simulink model "AGTF30SysDyn_PExPIn"  (R2023b)
settings: Solver=ode4  StartTime=0.0  StopTime=MWS.In.tend  FixedStep=MWS.In.Ts  RelTol=1e-3  EnableMultiTasking=on
model workspace: external: MAT-File (data not in the file)
values from neighbouring files (symbols this model uses):
  MWS = setup_initialize(MWS,startPt,SSsolverSP)    [Setup_Simulation.m]    (also in run_AGTF30e_script.m = Setup_Simulation(inputMethod,MWS.In,filename,Mdl,SSsolverSP))
undefined symbols (not defined in the file or in its folder): DiscIntNeverNeededParam
libraries: simulink x32, Lib_Solve_ModelSource_TMATS x28, Lib_EMTAT x27, Lib_Cntrl_FirstOrderSensor_TMATS x19, Lib_Cntrl_FirstOrderActuator_TMATS x2, Lib_Cntrl_LimitSelect_TMATS x2, Lib_Solve_OuterLoopIntegrator_TMATS x2, Lib_Cntrl_CorrectedSpeed_TMATS x1, Lib_Solve_IterNRSolverJC_TMATS x1, slpidlib x1
(part 4 of 8)

== system AGTF30SysDyn_PExPIn/Control System/Wf Controller/Controller/Set-Points ==
  Nominal SP : Inport
  N1cSP Limit SPs : Inport  Port=2
  Wf Limit SPs : Inport  Port=3
  Bus Creator : BusCreator  Inputs=3
  Bus Creator1 : BusCreator  Inputs=7
  Bus Creator2 : BusCreator  Inputs=3
  Demux : Demux  Outputs=7
  Demux1 : Demux  Outputs=3
  SPs : Outport  VectorParamsAs1DForOutWhenUnconnected=off
  wires:
  Nominal SP/1 -> Bus Creator/1  "N1c"
  N1cSP Limit SPs/1 -> Demux/1
  Bus Creator/1 -> SPs/1
  Demux/1 -> Bus Creator1/1  "T3Max"
  Demux/2 -> Bus Creator1/2  "T4Max"
  Demux/3 -> Bus Creator1/3  "T45Max"
  Demux/4 -> Bus Creator1/4  "N1Max"
  Demux/5 -> Bus Creator1/5  "N3Max"
  Demux/6 -> Bus Creator1/6  "Ps3Max"
  Demux/7 -> Bus Creator1/7  "Ps3Min"
  Bus Creator1/1 -> Bus Creator/2  "N1cSPLims"
  Bus Creator2/1 -> Bus Creator/3  "WfLims"
  Demux1/1 -> Bus Creator2/1  "Accel"
  Demux1/2 -> Bus Creator2/2  "Decel"
  Demux1/3 -> Bus Creator2/3  "WfMin"
  Wf Limit SPs/1 -> Demux1/1

== system AGTF30SysDyn_PExPIn/Control System/Wf Controller/Controller/Wf Limit Controllers ==
  note: ENABLE MIN FUEL FLOW LIMIT WHEN DECEL LIMIT IS NOT IN USE
  Alt : Inport
  MN : Inport  Port=2
  Wfmin : Inport  Port=3
  Wfmax : Inport  Port=4
  Wfcmd : Inport  Port=5
  phiEPT : Inport  Port=6
  phiBoost : Inport  Port=7
  N1cN : Inport  Port=8
  ps3 : Inport  Port=9
  RegNum : Inport  Port=10
  Accel Controller : Subsystem
  Compare To Constant : simulink/Logic and Bit Operations/Compare To Constant  relop=~=  const=7  OutDataTypeStr=boolean
  Decel Controller : Subsystem
  Divide : Product  Inputs=**
  Gain : Gain  Gain=0.95
  Memory : Memory
  Mux : Mux  Inputs=3
  Wf Accel : Outport  VectorParamsAs1DForOutWhenUnconnected=off
  Wf Decel : Outport  Port=2  VectorParamsAs1DForOutWhenUnconnected=off
  Wf Min : Outport  Port=3  VectorParamsAs1DForOutWhenUnconnected=off
  SPs : Outport  Port=4  VectorParamsAs1DForOutWhenUnconnected=off
  wires:
  Alt/1 -> Decel Controller/1(Alt), Accel Controller/1(Alt)
  Wfmax/1 -> Accel Controller/6(Wfmax)
  Decel Controller/2(WfminDecel_SP) -> Mux/2  "WfMinDecel"
  Accel Controller/2(WfmaxAccel_SP) -> Mux/1  "WfMaxAccel"
  Wfcmd/1 -> Accel Controller/7(Wfcmd), Decel Controller/7(Wf)
  Wfmin/1 -> Gain/1, Decel Controller/6(Wfmin)
  Decel Controller/1(Wfdmd) -> Wf Decel/1
  Accel Controller/1(Wfdmd) -> Wf Accel/1
  Mux/1 -> SPs/1
  MN/1 -> Decel Controller/2(MN), Accel Controller/2(MN)
  phiEPT/1 -> Decel Controller/4(phiEPT), Accel Controller/4(phiEPT)
  phiBoost/1 -> Decel Controller/5(phiBoost), Accel Controller/5(phiBoost)
  ps3/1 -> Accel Controller/8(ps3), Decel Controller/8(ps3)
  N1cN/1 -> Decel Controller/3(N1cN), Accel Controller/3(N1cN)
  Gain/1 -> Divide/1  "WfMin"
  Compare To Constant/1 -> Divide/2
  Divide/1 -> Mux/3, Wf Min/1
  RegNum/1 -> Memory/1
  Memory/1 -> Compare To Constant/1

== system AGTF30SysDyn_PExPIn/Control System/Wf Controller/Controller/Wf Limit Select ==
  WfReq : Inport
  Limits : Inport  Port=2
  Limit Selection : Lib_Cntrl_LimitSelect_TMATS/Limit Selection  SelectVec_M=MWS.Cntrl.WfCntrl.WfLim.Type  LimitsEn_M=MWS.Cntrl.WfCntrl.WfLim.En
  Wfdmd : Outport  VectorParamsAs1DForOutWhenUnconnected=off
  RegNum : Outport  Port=2  VectorParamsAs1DForOutWhenUnconnected=off
  wires:
  WfReq/1 -> Limit Selection/1
  Limits/1 -> Limit Selection/2
  Limit Selection/1 -> Wfdmd/1
  Limit Selection/2 -> RegNum/1

== system AGTF30SysDyn_PExPIn/EngineSystem/Power System/Electrical Power System/EM Variant Subsystem ==
  Vs [V] : Inport
  NemL [rpm] : Inport  Port=2
  TrqEML [ft-lb] : Inport  Port=3
  NemH [rpm] : Inport  Port=4
  TrqEMH [ft-lb] : Inport  Port=5
  NemS [rpm] : Inport  Port=6
  TrqEMS [ft-lb] : Inport  Port=7
  NemR [rpm] : Inport  Port=8
  TrqEMR [ft-lb] : Inport  Port=9
  NemC [rpm] : Inport  Port=10
  TrqEMC [ft-lb] : Inport  Port=11
  NemP [rpm] : Inport  Port=12
  TrqEMP [ft-lb] : Inport  Port=13
  Scalar DEM Subsystem : Subsystem  VariantControl=MWS.In.Options.EngineEMInt == 1
  Scalar PGB EM Subsystem : Subsystem  VariantControl=MWS.In.Options.EngineEMInt == 2
  Io [A] : Outport
  Out_LPEMbranch : Outport  Port=2
  Out_HPEMbranch : Outport  Port=3
  Out_SEMbranch : Outport  Port=4
  Out_REMbranch : Outport  Port=5
  Out_CEMbranch : Outport  Port=6
  Out_PEMbranch : Outport  Port=7

== system AGTF30SysDyn_PExPIn/EngineSystem/Power System/Electrical Power System/Energy Storage Subsystem ==
  I_2 [A] : Inport
  Load [hp] : Inport  Port=2
  Bus Creator : BusCreator  Inputs=9
  Bus Selector : BusSelector  OutputSignals=P_1; W,P_2; W
  Bus Selector1 : BusSelector  OutputSignals=P_2; W,I; A
  Bus Selector2 : BusSelector  OutputSignals=I; A
  Cable : Lib_EMTAT/Components/Power Flow/Cable  R=MWS.EPS.Cable.R
      settings: AttributesFormatString=Cable  SourceProductName=EMTAT
  Constant1 : Constant  Value=0
  Constant2 : Constant  Value=0
  Current Junction : Lib_EMTAT/Components/Power Flow/Current Junction  Nb=1
      settings: AttributesFormatString=Current Junction  SourceProductName=EMTAT
  Current Junction1 : Lib_EMTAT/Components/Power Flow/Current Junction  Nb=1
      settings: AttributesFormatString=Current Junction  SourceProductName=EMTAT
  DCDC Variant Subsystem : Subsystem  Variant=on
  ESD Variant Subsystem : Subsystem  Variant=on
  Mux : Mux  Inputs=2
  Resistive Load Bank : Lib_EMTAT/Components/Power Flow/Resistive Load Bank
      settings: AttributesFormatString=Resistive Load Bank  SourceProductName=EMTAT
  Sum1 : Sum  Inputs=+|+
  Terminator1 : Terminator
  Terminator2 : Terminator
  Unit Delay : UnitDelay  InitialCondition=MWS.EPS.Cable.Iout_IC  SampleTime=-1  HasFrameUpgradeWarning=on
  hp to W : Gain  Gain=745.7
  V_DC_Out [V] : Outport
  Out_SupplySys : Outport  Port=2
  SoC [%] : Outport  Port=3
  wires:
  Sum1/1 -> [ESD_Pwr]
  Bus Selector1/1 -> [SuppCable_Pwr], Sum1/1  "<P_2; W>"
  Unit Delay/1 -> Cable/4
  Bus Selector/2 -> [DCDC_Pwr]  "<P_2; W>"
  Cable/1 -> DCDC Variant Subsystem/1(V_ESD [V])
  ESD Variant Subsystem/2(SoC [%]) -> SoC [%]/1
  Load [hp]/1 -> hp to W/1
  DCDC Variant Subsystem/3(Outputs) -> Bus Selector/1
  I_2 [A]/1 -> Current Junction1/1, Mux/1
  Bus Selector/1 -> [Bus_Pwr]  "<P_1; W>"
  Cable/3 -> Terminator1/1
  Cable/5 -> Unit Delay/1
  Constant1/1 -> Cable/3
  DCDC Variant Subsystem/2(Vo [V]) -> [V_Bus], V_DC_Out [V]/1, Resistive Load Bank/1
  Cable/2 -> Bus Selector1/1
  Bus Creator/1 -> Out_SupplySys/1
  [DCDC_Pwr] -> Bus Creator/2  "DCDC_Pwr"
  [Bus_Pwr] -> Bus Creator/1  "Bus_Pwr"
  [ESD_Pwr] -> Bus Creator/4  "ESD_Pwr"
  [SuppCable_Pwr] -> Bus Creator/3  "SuppCable_Pwr"
  DCDC Variant Subsystem/1(Io [A]) -> Cable/2
  Cable/4 -> ESD Variant Subsystem/1(I [A])
  ESD Variant Subsystem/1(Vo [V]) -> [V_ESD], Cable/1
  Resistive Load Bank/3 -> Mux/2
  Resistive Load Bank/1 -> Bus Selector2/1
  Resistive Load Bank/2 -> Terminator2/1
  Constant2/1 -> Resistive Load Bank/3
  Mux/1 -> Current Junction/1
  Current Junction/1 -> DCDC Variant Subsystem/2(I_Bus [A])
  hp to W/1 -> Sum1/2, Resistive Load Bank/2
  Bus Selector1/2 -> [I_ESD]  "<I; A>"
  Bus Selector2/1 -> [I_Load]  "<I; A>"
  [V_Bus] -> Bus Creator/5  "V_Bus"
  [V_ESD] -> Bus Creator/6  "V_ESD"
  [I_Bus] -> Bus Creator/7  "I_Bus"
  [I_Load] -> Bus Creator/8  "I_Load"
  [I_ESD] -> Bus Creator/9  "I_ESD"
  Current Junction1/1 -> [I_Bus]

== system AGTF30SysDyn_PExPIn/Control System/Electric Machine Controllers/EM Controllers/DEM Control/DEM EM Controllers ==
  note: The load is the electrical power demand from the bus needed for sustaining engine and aircraft subsystems (PExAC) and extraneous propulsive loads (in the case of PEx mode). In the case of PEx mode, the electrical load is modified to essentially match the power extraction commanded for the electric machines. "Essentially" is used because it won't match actually given cable losses. So the SOC controller will need to make up a slight difference.
  PwrInLPEMNomMan : Inport
  PwrInLPEMNomManEn : Inport  Port=2
  PwrInLPEMOffNomMan : Inport  Port=3
  PwrInLPEMOffNomManEn : Inport  Port=4
  PwrInHPEMNomMan : Inport  Port=5
  PwrInHPEMNomManEn : Inport  Port=6
  PwrInHPEMOffNomMan : Inport  Port=7
  PwrInHPEMOffNomManEn : Inport  Port=8
  PwrInLP_Base : Inport  Port=9
  PwrInHP_Base : Inport  Port=10
  NemL : Inport  Port=11
  NemH : Inport  Port=12
  PwrEPT : Inport  Port=13
  PwrInAccel_TEEM : Inport  Port=14
  PwrExAccel_TEEM : Inport  Port=15
  PwrXDecel_TEEM : Inport  Port=16
  PwrCharge : Inport  Port=17
  PExAC : Inport  Port=18
  PwrSys : Inport  Port=19
  EMH Controller : Subsystem
  EML Controller : Subsystem
  EPT Pwr Calc : Subsystem
  Sum : Sum  Inputs=+|+
  PwrEML : Outport
  PwrEMH : Outport  Port=2
  TrqEML : Outport  Port=3
  TrqEMH : Outport  Port=4
  PwrLoad : Outport  Port=5
  wires:
  NemH/1 -> EMH Controller/6(NemH)
  PwrInAccel_TEEM/1 -> EMH Controller/8(PwrInAccel_TEEM)
  EML Controller/2(TrqEML) -> TrqEML/1
  EMH Controller/2(TrqEMH) -> TrqEMH/1
  PwrInLP_Base/1 -> EML Controller/5(PwrInLP_Base)
  PwrInHP_Base/1 -> EMH Controller/5(PwrInHP_Base)
  PwrInLPEMOffNomManEn/1 -> EML Controller/4(PwrInLPEMOffNomManEn)
  NemL/1 -> EML Controller/6(NemL)
  PwrInLPEMNomMan/1 -> EML Controller/1(PwrInLPEMNomMan)
  PwrInHPEMOffNomMan/1 -> EMH Controller/3(PwrInHPEMOffNomMan)
  PwrInHPEMNomManEn/1 -> EMH Controller/2(PwrInHPEMNomManEn)
  EML Controller/1(PwrEML) -> PwrEML/1
  PwrInLPEMNomManEn/1 -> EML Controller/2(PwrInLPEMNomManEn)
  PwrInHPEMOffNomManEn/1 -> EMH Controller/4(PwrInHPEMOffNomManEn)
  PwrInLPEMOffNomMan/1 -> EML Controller/3(PwrInLPEMOffNomMan)
  PwrInHPEMNomMan/1 -> EMH Controller/1(PwrInHPEMNomMan)
  EMH Controller/1(PwrEMH) -> PwrEMH/1
  PwrXDecel_TEEM/1 -> EMH Controller/9(PwrXDecel_TEEM), EML Controller/9(PwrXDecel_TEEM)
  PwrEPT/1 -> EPT Pwr Calc/1(PwrEPT)
  EPT Pwr Calc/1(PwrEML_EPT) -> EML Controller/7(PwrInLPEPT)
  EPT Pwr Calc/2(PwrEMH_EPT) -> EMH Controller/7(PwrInHPEPT)
  Sum/1 -> PwrLoad/1
  PwrCharge/1 -> EMH Controller/10(PwrCharge)
  PwrExAccel_TEEM/1 -> EML Controller/8(PwrExAccel_TEEM)
  PwrSys/1 -> EMH Controller/11(PwrSys), EML Controller/10(PwrSys)
  PExAC/1 -> EMH Controller/12(PExAC)
  EML Controller/3(PwrLoadL) -> [PwrLoadL]
  EMH Controller/3(PwrLoadEMH) -> [PwrLoadH]
  [PwrLoadL] -> Sum/1
  [PwrLoadH] -> Sum/2

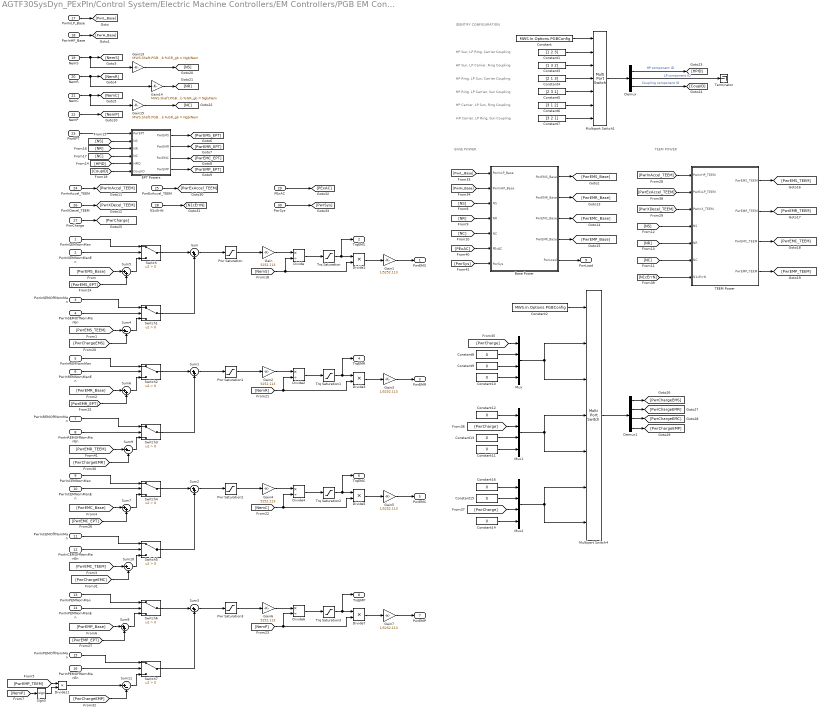
== system AGTF30SysDyn_PExPIn/Control System/Electric Machine Controllers/EM Controllers/PGB EM Control/VEATE EM Controllers ==
  note: HP Sun, LP RIng, Carrier Coupling
  note: HP Sun, LP Carrier, Ring Coupling
  note: IDENTIFY CONFIGURATION
  note: HP Ring, LP Sun, Carrier Coupling
  note: HP Carrier, LP Sun, Ring Coupling
  note: HP Ring, LP Carrier, Sun Coupling
  note: HP Carrier, LP Ring, Sun Coupling
  note: TEEM POWER
  note: BASE POWER
  PwrInSEMNomMan : Inport
  PwrInSEMNomManEn : Inport  Port=2
  PwrInSEMOffNomMan : Inport  Port=3
  PwrInSEMOffNomManEn : Inport  Port=4
  PwrInREMNomMan : Inport  Port=5
  PwrInREMNomManEn : Inport  Port=6
  PwrInREMOffNomMan : Inport  Port=7
  PwrInREMOffNomManEn : Inport  Port=8
  PwrInCEMNomMan : Inport  Port=9
  PwrInCEMNomManEn : Inport  Port=10
  PwrInCEMOffNomMan : Inport  Port=11
  PwrInCEMOffNomManEn : Inport  Port=12
  PwrInPEMNomMan : Inport  Port=13
  PwrInPEMNomManEn : Inport  Port=14
  PwrInPEMOffNomMan : Inport  Port=15
  PwrInPEMOffNomManEn : Inport  Port=16
  PwrInLP_Base : Inport  Port=17
  PwrInHP_Base : Inport  Port=18
  NemS : Inport  Port=19
  NemR : Inport  Port=20
  NemC : Inport  Port=21
  NemP : Inport  Port=22
  PwrEPT : Inport  Port=23
  PwrInAccel_TEEM : Inport  Port=24
  PwrExAccel_TEEM : Inport  Port=25
  PwrXDecel_TEEM : Inport  Port=26
  PwrCharge : Inport  Port=27
  N1cErrN : Inport  Port=28
  PExAC : Inport  Port=29
  PwrSys : Inport  Port=30
  Base Power : Subsystem
  Constant : Constant  Value=MWS.In.Options.PGBConfig
  Constant1 : Constant  Value=[1 2 3]
  Constant{8..16} (9 alike) : Constant  Value=0
  Constant2 : Constant  Value=MWS.In.Options.PGBConfig
  Constant3 : Constant  Value=[1 3 2]
  Constant4 : Constant  Value=[2 1 3]
  Constant5 : Constant  Value=[2 3 1]
  Constant6 : Constant  Value=[3 1 2]
  Constant7 : Constant  Value=[3 2 1]
  Demux : Demux  Outputs=3
  Demux1 : Demux
  Divide{,2,4,6} (4 alike) : Product  Inputs=*/
  Divide{1,3,5,7,11} (5 alike) : Product  Inputs=**
  EPT Powers : Subsystem
  Gain{,2,4,6} (4 alike) : Gain  Gain=5252.113
  Gain{1,3,5,7} (4 alike) : Gain  Gain=1/5252.113
  Gain13 : Gain  Gain=MWS.Shaft.PGB.Sun.GR_gb %GR_gb = Ngb/Nem
  Gain14 : Gain  Gain=MWS.Shaft.PGB.Ring.GR_gb %GR_gb = Ngb/Nem
  Gain15 : Gain  Gain=MWS.Shaft.PGB.Carrier.GR_gb %GR_gb = Ngb/Nem
  Multiport Switch1 : MultiPortSwitch  Inputs=6  SaturateOnIntegerOverflow=off  InputSameDT=off
  Multiport Switch4 : MultiPortSwitch  Inputs=6  SaturateOnIntegerOverflow=off  InputSameDT=off
  Mux : Mux
  Mux1 : Mux
  Mux2 : Mux
  Pwr Saturation : Saturate  UpperLimit=MWS.PowerSystem.EMS.PMax  LowerLimit=-MWS.PowerSystem.EMS.PMax
  Pwr Saturation1 : Saturate  UpperLimit=MWS.PowerSystem.EMR.PMax  LowerLimit=-MWS.PowerSystem.EMR.PMax
  Pwr Saturation2 : Saturate  UpperLimit=MWS.PowerSystem.EMC.PMax  LowerLimit=-MWS.PowerSystem.EMC.PMax
  Pwr Saturation3 : Saturate  UpperLimit=MWS.PowerSystem.EMP.PMax  LowerLimit=-MWS.PowerSystem.EMP.PMax
  Sign3 : Signum
  Sum{,1..3,5..8} (8 alike) : Sum  Inputs=|++
  Sum{4,9..11} (4 alike) : Sum  Inputs=|+-
  Switch{,1..7} (8 alike) : Switch  Criteria=u2 > Threshold  SaturateOnIntegerOverflow=off  InputSameDT=off
  TEEM Power : Subsystem
  Terminator : Terminator
  Trq Saturation : Saturate  UpperLimit=MWS.PowerSystem.EMS.TrqMax  LowerLimit=-MWS.PowerSystem.EMS.TrqMax
  Trq Saturation1 : Saturate  UpperLimit=MWS.PowerSystem.EMR.TrqMax  LowerLimit=-MWS.PowerSystem.EMR.TrqMax
  Trq Saturation2 : Saturate  UpperLimit=MWS.PowerSystem.EMC.TrqMax  LowerLimit=-MWS.PowerSystem.EMC.TrqMax
  Trq Saturation3 : Saturate  UpperLimit=MWS.PowerSystem.EMP.TrqMax  LowerLimit=-MWS.PowerSystem.EMP.TrqMax
  PwrEMS : Outport
  TrqEMS : Outport  Port=2
  PwrEMR : Outport  Port=3
  TrqEMR : Outport  Port=4
  PwrEMC : Outport  Port=5
  TrqEMC : Outport  Port=6
  PwrEMP : Outport  Port=7
  TrqEMP : Outport  Port=8
  PwrLoad : Outport  Port=9
  wires:
  PwrInSEMNomManEn/1 -> Switch/2
  PwrInSEMNomMan/1 -> Switch/1
  Switch/1 -> Sum/1
  Switch1/1 -> Sum/2
  PwrInSEMOffNomManEn/1 -> Switch1/2
  PwrInSEMOffNomMan/1 -> Switch1/1
  Sum/1 -> Pwr Saturation/1
  Pwr Saturation/1 -> Gain/1
  Gain/1 -> Divide/1
  [NemS] -> Divide/2, Divide1/2
  Divide/1 -> Trq Saturation/1
  Trq Saturation/1 -> Divide1/1, TrqEMS/1
  Divide1/1 -> Gain1/1
  Gain1/1 -> PwrEMS/1
  PwrInAccel_TEEM/1 -> [PwrInAccel_TEEM]
  PwrInLP_Base/1 -> [PwrL_Base]
  PwrInHP_Base/1 -> [PwrH_Base]
  [PwrEMS_Base] -> Sum5/1
  Sum1/1 -> Pwr Saturation1/1
  Switch3/1 -> Sum1/2
  PwrInREMOffNomManEn/1 -> Switch3/2
  [PwrEMR_TEEM] -> Sum9/1
  [PwrEMR_Base] -> Sum6/1
  Divide3/1 -> Gain3/1
  [NemR] -> Divide2/2, Divide3/2
  Pwr Saturation1/1 -> Gain2/1
  Gain2/1 -> Divide2/1
  PwrInREMNomMan/1 -> Switch2/1
  Switch2/1 -> Sum1/1
  Divide2/1 -> Trq Saturation1/1
  Gain3/1 -> PwrEMR/1
  PwrInREMOffNomMan/1 -> Switch3/1
  Trq Saturation1/1 -> TrqEMR/1, Divide3/1
  PwrInREMNomManEn/1 -> Switch2/2
  Sum2/1 -> Pwr Saturation2/1
  Switch5/1 -> Sum2/2
  PwrInCEMOffNomManEn/1 -> Switch5/2
  [PwrEMC_Base] -> Sum7/1
  Divide5/1 -> Gain5/1
  [NemC] -> Divide5/2, Divide4/2
  Pwr Saturation2/1 -> Gain4/1
  Gain4/1 -> Divide4/1
  PwrInCEMNomMan/1 -> Switch4/1
  Switch4/1 -> Sum2/1
  Divide4/1 -> Trq Saturation2/1
  Gain5/1 -> PwrEMC/1
  PwrInCEMOffNomMan/1 -> Switch5/1
  Trq Saturation2/1 -> TrqEMC/1, Divide5/1
  PwrInCEMNomManEn/1 -> Switch4/2
  Sum3/1 -> Pwr Saturation3/1
  Switch7/1 -> Sum3/2
  PwrInPEMOffNomManEn/1 -> Switch7/2
  Divide11/1 -> Sum11/1
  [PwrEMP_Base] -> Sum8/1
  Divide7/1 -> Gain7/1
  [NemP] -> Divide7/2, Divide6/2
  Pwr Saturation3/1 -> Gain6/1
  Gain6/1 -> Divide6/1
  PwrInPEMNomMan/1 -> Switch6/1
  Switch6/1 -> Sum3/1
  Divide6/1 -> Trq Saturation3/1
  Gain7/1 -> PwrEMP/1
  PwrInPEMOffNomMan/1 -> Switch7/1
  Trq Saturation3/1 -> TrqEMP/1, Divide7/1
  PwrInPEMNomManEn/1 -> Switch6/2
  NemS/1 -> Gain13/1, [NemS]
  NemC/1 -> Gain15/1, [NemC]
  NemP/1 -> [NemP]
  [NC] -> EPT Powers/4(NC)
  [NR] -> EPT Powers/3(NR)
  [NS] -> EPT Powers/2(NS)
  PwrEPT/1 -> EPT Powers/1(PwrEPT)
  EPT Powers/1(PwrEMS) -> [PwrEMS_EPT]
  EPT Powers/2(PwrEMR) -> [PwrEMR_EPT]
  EPT Powers/3(PwrEMC) -> [PwrEMC_EPT]
  EPT Powers/4(PwrEMP) -> [PwrEMP_EPT]
  PwrXDecel_TEEM/1 -> [PwrXDecel_TEEM]
  Sum5/1 -> Switch/3
  [PwrEMS_EPT] -> Sum5/2
  Sum6/1 -> Switch2/3
  Sum7/1 -> Switch4/3
  Sum8/1 -> Switch6/3
  [PwrEMR_EPT] -> Sum6/2
  [PwrEMC_EPT] -> Sum7/2
  [PwrEMP_EPT] -> Sum8/2
  Gain13/1 -> [NS]
  Gain15/1 -> [NC]
  NemR/1 -> Gain14/1, [NemR]
  Gain14/1 -> [NR]
  Base Power/1(PwrEMS_Base) -> [PwrEMS_Base]
  Base Power/2(PwrEMR_Base) -> [PwrEMR_Base]
  Base Power/3(PwrEMC_Base) -> [PwrEMC_Base]
  Base Power/4(PwrEMP_Base) -> [PwrEMP_Base]
  [NC] -> Base Power/5(NC)
  [NR] -> Base Power/4(NR)
  [NS] -> Base Power/3(NS)
  [PwrH_Base] -> Base Power/2(PwrInHP_Base)
  [PwrL_Base] -> Base Power/1(PwrInLP_Base)
  [PwrInAccel_TEEM] -> TEEM Power/1(PwrInHP_TEEM)
  [PwrXDecel_TEEM] -> TEEM Power/3(PwrInX_TEEM)
  [NS] -> TEEM Power/4(NS)
  [NR] -> TEEM Power/5(NR)
  [NC] -> TEEM Power/6(NC)
  TEEM Power/1(PwrEMS_TEEM) -> [PwrEMS_TEEM]
  TEEM Power/2(PwrEMR_TEEM) -> [PwrEMR_TEEM]
  TEEM Power/3(PwrEMC_TEEM) -> [PwrEMC_TEEM]
  TEEM Power/4(PwrEMP_TEEM) -> [PwrEMP_TEEM]
  Demux/3 -> [CoupID]  "Coupling component ID"
  Demux/2 -> Terminator/1  "LP component ID"
  Constant5/1 -> Multiport Switch1/5
  Constant6/1 -> Multiport Switch1/6
  Multiport Switch1/1 -> Demux/1
  Constant1/1 -> Multiport Switch1/2
  Constant7/1 -> Multiport Switch1/7
  Constant/1 -> Multiport Switch1/1
  Constant3/1 -> Multiport Switch1/3
  Constant4/1 -> Multiport Switch1/4
  Demux/1 -> [HPID]  "HP component ID"
  [HPID] -> EPT Powers/5(HPID)
  [CoupID] -> EPT Powers/6(CoupID)
  PwrCharge/1 -> [PwrCharge]
  Base Power/5(PwrLoad) -> PwrLoad/1
  Sum4/1 -> Switch1/3
  [PwrChargeEMS] -> Sum4/2
  [PwrChargeEMR] -> Sum9/2
  [PwrChargeEMC] -> Sum10/2
  [PwrChargeEMP] -> Sum11/2
  Sum9/1 -> Switch3/3
  Sum10/1 -> Switch5/3
  Sum11/1 -> Switch7/3
  Constant2/1 -> Multiport Switch4/1
  Multiport Switch4/1 -> Demux1/1
  [PwrCharge] -> Mux/1
  Constant8/1 -> Mux/2
  Constant9/1 -> Mux/3
  Constant10/1 -> Mux/4
  Demux1/1 -> [PwrChargeEMS]
  Demux1/2 -> [PwrChargeEMR]
  Demux1/3 -> [PwrChargeEMC]
  Demux1/4 -> [PwrChargeEMP]
  Mux/1 -> Multiport Switch4/2, Multiport Switch4/3
  Constant11/1 -> Mux1/4
  [PwrCharge] -> Mux1/2
  Constant12/1 -> Mux1/1
  Constant13/1 -> Mux1/3
  Mux1/1 -> Multiport Switch4/5, Multiport Switch4/4
  Constant14/1 -> Mux2/4
  [PwrCharge] -> Mux2/3
  Constant15/1 -> Mux2/2
  Constant16/1 -> Mux2/1
  Mux2/1 -> Multiport Switch4/6, Multiport Switch4/7
  PwrExAccel_TEEM/1 -> [PwrExAccel_TEEM]
  [PwrExAccel_TEEM] -> TEEM Power/2(PwrExLP_TEEM)
  N1cErrN/1 -> [N1cErrN]
  [N1cErrN] -> TEEM Power/7(N1cErrN)
  [PwrEMS_TEEM] -> Sum4/1
  [PwrEMC_TEEM] -> Sum10/1
  [PwrEMP_TEEM] -> Divide11/1
  [NemP] -> Sign3/1
  Sign3/1 -> Divide11/2
  [PExAC] -> Base Power/6(PExAC)
  [PwrSys] -> Base Power/7(PwrSys)
  PExAC/1 -> [PExAC]
  PwrSys/1 -> [PwrSys]

== system AGTF30SysDyn_PExPIn/Control System/Scheduling/Steady State EM Power - MaxMin/HP and LP Pwr Calc/Gearbox Speeds ==
  k_Alt : Inport
  f_Alt : Inport  Port=2
  k_MN : Inport  Port=3
  f_MN : Inport  Port=4
  PwrBase_LP : Inport  Port=5
  PwrBase_HP : Inport  Port=6
  PwrEPT_LPg : Inport  Port=7
  PwrEPT_HPg : Inport  Port=8
  Constant35 : Constant  Value=[[0:1:length(MWS.Cntrl.SPSched.PL_vec)-2],length(MWS.Cntrl.SPSched.PL_vec)-2]
  Constant36 : Constant  Value=[zeros(1,length(MWS.Cntrl.SPSched.PL_vec)-1),1]
  Mux12 : Mux  Inputs=2
  N2 Interpolation Using Prelookup : Interpolation_n-D  NumberOfTableDimensions=5  Table=MWS.Cntrl.Sched.N2.N2_array  InternalRulePriority=Speed
      settings: InputPortMap=u0,u1,u2,u3,u4,u5,u6,u7,u8,u9
  N2min Lookup Table Dynamic : simulink/Lookup Tables/Lookup Table Dynamic  LookUpMeth=Interpolation-Use End Values  OutDataType=fixdt('double')  OutScaling=[]  OutputDataTypeScalingMode=Specify via dialog  OutDataTypeStr=double  DoSatur=off
  N3 Interpolation Using Prelookup : Interpolation_n-D  NumberOfTableDimensions=5  Table=MWS.Cntrl.Sched.N3.N3_array  InternalRulePriority=Speed
      settings: InputPortMap=u0,u1,u2,u3,u4,u5,u6,u7,u8,u9
  N3min Lookup Table Dynamic : simulink/Lookup Tables/Lookup Table Dynamic  LookUpMeth=Interpolation-Use End Values  OutDataType=fixdt('double')  OutScaling=[]  OutputDataTypeScalingMode=Specify via dialog  OutDataTypeStr=double  DoSatur=off
  Ps3 Interpolation Using Prelookup : Interpolation_n-D  NumberOfTableDimensions=5  Table=MWS.Cntrl.Sched.Ps3.Ps3_array  InternalRulePriority=Speed
      settings: InputPortMap=u0,u1,u2,u3,u4,u5,u6,u7,u8,u9
  Ps3min Interpolation Using Prelookup : Interpolation_n-D  Table=MWS.Cntrl.Sched.Ps3Min.Ps3Min_array  InterpMethod=Linear Lagrange  InternalRulePriority=Speed
  PwrInHP Prelookup : PreLookup  BreakpointsData=MWS.Cntrl.SPSched.PwrInHP_vec  IndexSearchMethod=Linear search  BeginIndexSearchUsingPreviousIndexResult=on  ExtrapMethod=Linear
  PwrInLP Prelookup : PreLookup  BreakpointsData=MWS.Cntrl.SPSched.PwrInLP_vec  IndexSearchMethod=Linear search  BeginIndexSearchUsingPreviousIndexResult=on  ExtrapMethod=Linear
  Spool to PGB speeds : Subsystem
  Sum : Sum  Inputs=|++
  Sum1 : Sum  Inputs=|++
  NPGB : Outport
  wires:
  [N3vec] -> N3min Lookup Table Dynamic/3
  Spool to PGB speeds/1(NPGB) -> NPGB/1
  [f_PwrInHP] -> N2 Interpolation Using Prelookup/10, N3 Interpolation Using Prelookup/10, Ps3 Interpolation Using Prelookup/10
  [f_PwrInLP] -> N2 Interpolation Using Prelookup/8, N3 Interpolation Using Prelookup/8, Ps3 Interpolation Using Prelookup/8
  [k_PwrInHP] -> N2 Interpolation Using Prelookup/9, N3 Interpolation Using Prelookup/9, Ps3 Interpolation Using Prelookup/9
  N2 Interpolation Using Prelookup/1 -> [N2vec]
  k_Alt/1 -> N2 Interpolation Using Prelookup/3, N3 Interpolation Using Prelookup/3, Ps3 Interpolation Using Prelookup/3, Ps3min Interpolation Using Prelookup/1
  PwrInLP Prelookup/1 -> [k_PwrInLP]  "k_PwrInHPMn"
  N3min Lookup Table Dynamic/1 -> Mux12/2  "N3min"
  f_MN/1 -> N2 Interpolation Using Prelookup/6, N3 Interpolation Using Prelookup/6, Ps3 Interpolation Using Prelookup/6, Ps3min Interpolation Using Prelookup/4
  PwrEPT_LPg/1 -> Sum/2
  k_MN/1 -> N2 Interpolation Using Prelookup/5, N3 Interpolation Using Prelookup/5, Ps3 Interpolation Using Prelookup/5, Ps3min Interpolation Using Prelookup/3
  Constant35/1 -> N3 Interpolation Using Prelookup/1, N2 Interpolation Using Prelookup/1, Ps3 Interpolation Using Prelookup/1
  PwrInHP Prelookup/1 -> [k_PwrInHP]  "k_PwrInHPMn"
  f_Alt/1 -> N2 Interpolation Using Prelookup/4, N3 Interpolation Using Prelookup/4, Ps3 Interpolation Using Prelookup/4, Ps3min Interpolation Using Prelookup/2
  [k_PwrInLP] -> N2 Interpolation Using Prelookup/7, N3 Interpolation Using Prelookup/7, Ps3 Interpolation Using Prelookup/7
  [Ps3vec] -> N2min Lookup Table Dynamic/2
  Sum1/1 -> PwrInHP Prelookup/1
  [Ps3vec] -> N3min Lookup Table Dynamic/2
  Constant36/1 -> N3 Interpolation Using Prelookup/2, N2 Interpolation Using Prelookup/2, Ps3 Interpolation Using Prelookup/2
  PwrBase_HP/1 -> Sum1/1
  PwrInHP Prelookup/2 -> [f_PwrInHP]  "f_PwrInHPMx"
  [Ps3min] -> N3min Lookup Table Dynamic/1
  Ps3 Interpolation Using Prelookup/1 -> [Ps3vec]
  [N2vec] -> N2min Lookup Table Dynamic/3
  Ps3min Interpolation Using Prelookup/1 -> [Ps3min]
  Sum/1 -> PwrInLP Prelookup/1
  PwrEPT_HPg/1 -> Sum1/2
  [Ps3min] -> N2min Lookup Table Dynamic/1
  N3 Interpolation Using Prelookup/1 -> [N3vec]
  PwrInLP Prelookup/2 -> [f_PwrInLP]  "f_PwrInHPMx"
  N2min Lookup Table Dynamic/1 -> Mux12/1  "N2min"
  Mux12/1 -> Spool to PGB speeds/1(N)
  PwrBase_LP/1 -> Sum/1

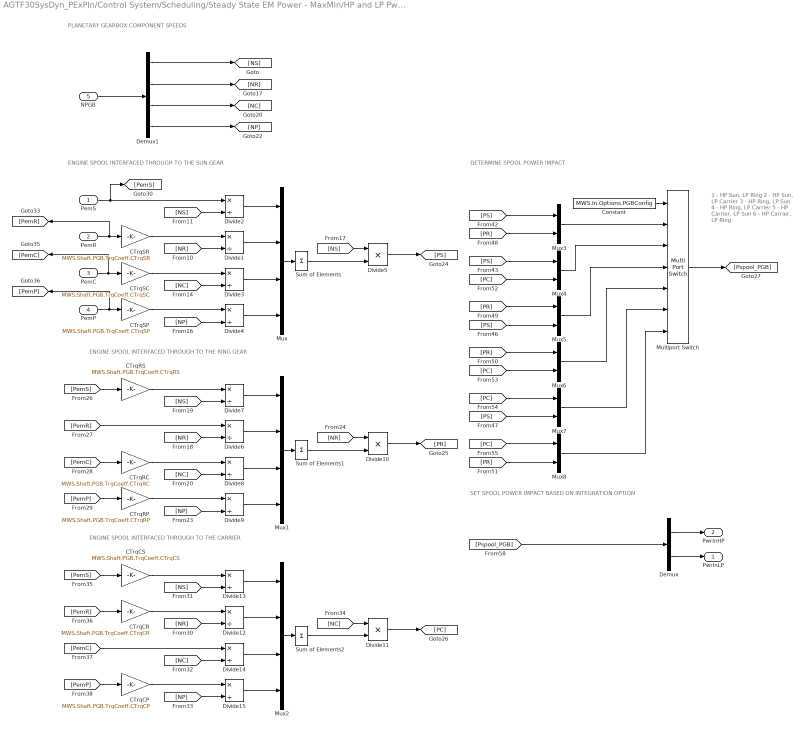
== system AGTF30SysDyn_PExPIn/Control System/Scheduling/Steady State EM Power - MaxMin/HP and LP Pwr Calc/Spool Power Impact ==
  note: 1 - HP Sun, LP Ring
      | 2 - HP Sun, LP Carrier
      | 3 - HP Ring, LP Sun
      | 4 - HP Ring, LP Carrier
      | 5 - HP Carrier, LP Sun
      | 6 - HP Carrier, LP Ring
  note: ENGINE SPOOL INTERFACED THROUGH TO THE SUN GEAR
  note: ENGINE SPOOL INTERFACED THROUGH TO THE RING GEAR
  note: ENGINE SPOOL INTERFACED THROUGH TO THE CARRIER
  note: DETERMINE SPOOL POWER IMPACT
  note: SET SPOOL POWER IMPACT BASED ON INTEGRATION OPTION
  note: PLANETARY GEARBOX COMPONENT SPEEDS
  PemS : Inport
  PemR : Inport  Port=2
  PemC : Inport  Port=3
  PemP : Inport  Port=4
  NPGB : Inport  Port=5
  CTrqCP : Gain  Gain=MWS.Shaft.PGB.TrqCoeff.CTrqCP
  CTrqCR : Gain  Gain=MWS.Shaft.PGB.TrqCoeff.CTrqCR
  CTrqCS : Gain  Gain=MWS.Shaft.PGB.TrqCoeff.CTrqCS
  CTrqRC : Gain  Gain=MWS.Shaft.PGB.TrqCoeff.CTrqRC
  CTrqRP : Gain  Gain=MWS.Shaft.PGB.TrqCoeff.CTrqRP
  CTrqRS : Gain  Gain=MWS.Shaft.PGB.TrqCoeff.CTrqRS
  CTrqSC : Gain  Gain=MWS.Shaft.PGB.TrqCoeff.CTrqSC
  CTrqSP : Gain  Gain=MWS.Shaft.PGB.TrqCoeff.CTrqSP
  CTrqSR : Gain  Gain=MWS.Shaft.PGB.TrqCoeff.CTrqSR
  Constant : Constant  Value=MWS.In.Options.PGBConfig
  Demux : Demux  Outputs=2
  Demux1 : Demux
  Divide{1..4,6..9,12..15} (12 alike) : Product  Inputs=*/
  Divide10 : Product  Inputs=**
  Divide11 : Product  Inputs=**
  Divide5 : Product  Inputs=**
  Multiport Switch : MultiPortSwitch  Inputs=6  SaturateOnIntegerOverflow=off  InputSameDT=off
  Mux : Mux
  Mux1 : Mux
  Mux2 : Mux
  Mux{3..8} (6 alike) : Mux  Inputs=2
  Sum of Elements : Sum  Inputs=+
  Sum of Elements1 : Sum  Inputs=+
  Sum of Elements2 : Sum  Inputs=+
  PwrInLP : Outport
  PwrInHP : Outport  Port=2
  wires:
  [PemP] -> CTrqRP/1
  CTrqRC/1 -> Divide8/1
  [NP] -> Divide4/2
  CTrqRP/1 -> Divide9/1
  [PemS] -> CTrqCS/1
  Mux8/1 -> Multiport Switch/7
  [NC] -> Divide14/2
  Mux5/1 -> Multiport Switch/4
  [PR] -> Mux5/1
  [NP] -> Divide15/2
  CTrqCS/1 -> Divide13/1
  CTrqCP/1 -> Divide15/1
  [PR] -> Mux3/2
  [PC] -> Mux8/1
  CTrqRS/1 -> Divide7/1
  Divide4/1 -> Mux/4
  [PS] -> Mux5/2
  [Pspool_PGB] -> Demux/1
  [NS] -> Divide7/2
  [PR] -> Mux8/2
  Divide11/1 -> [PC]
  Divide7/1 -> Mux1/1
  CTrqSR/1 -> Divide1/1
  Divide14/1 -> Mux2/3
  [PemC] -> Divide14/1
  [PemC] -> CTrqRC/1
  Mux4/1 -> Multiport Switch/3
  [PC] -> Mux4/2
  [NP] -> Divide9/2
  CTrqSC/1 -> Divide3/1
  Divide2/1 -> Mux/1
  Mux2/1 -> Sum of Elements2/1
  PemR/1 -> [PemR], CTrqSR/1
  [NR] -> Divide12/2
  Divide15/1 -> Mux2/4
  Divide8/1 -> Mux1/3
  [NS] -> Divide2/2
  [PC] -> Mux6/2
  Constant/1 -> Multiport Switch/1
  [PemP] -> CTrqCP/1
  Divide10/1 -> [PR]
  [NC] -> Divide11/1
  Divide3/1 -> Mux/3
  [NS] -> Divide5/1
  Divide13/1 -> Mux2/1
  [NS] -> Divide13/2
  [NR] -> Divide1/2
  Mux6/1 -> Multiport Switch/5
  Divide5/1 -> [PS]
  Divide12/1 -> Mux2/2
  PemP/1 -> [PemP], CTrqSP/1
  [PS] -> Mux3/1
  [NR] -> Divide10/1
  [PR] -> Mux6/1
  PemS/1 -> [PemS], Divide2/1
  [PemS] -> CTrqRS/1
  [NC] -> Divide3/2
  CTrqSP/1 -> Divide4/1
  Mux7/1 -> Multiport Switch/6
  CTrqCR/1 -> Divide12/1
  Divide1/1 -> Mux/2
  [PemR] -> CTrqCR/1
  PemC/1 -> [PemC], CTrqSC/1
  [PC] -> Mux7/1
  [PS] -> Mux7/2
  [PS] -> Mux4/1
  Multiport Switch/1 -> [Pspool_PGB]
  [PemR] -> Divide6/1
  Mux3/1 -> Multiport Switch/2
  [NC] -> Divide8/2
  Divide9/1 -> Mux1/4
  Mux1/1 -> Sum of Elements1/1
  Divide6/1 -> Mux1/2
  [NR] -> Divide6/2
  Mux/1 -> Sum of Elements/1
  Demux/1 -> PwrInHP/1
  Demux/2 -> PwrInLP/1
  NPGB/1 -> Demux1/1
  Demux1/1 -> [NS]
  Demux1/2 -> [NR]
  Demux1/3 -> [NC]
  Demux1/4 -> [NP]
  Sum of Elements/1 -> Divide5/2
  Sum of Elements1/1 -> Divide10/2
  Sum of Elements2/1 -> Divide11/2

== system AGTF30SysDyn_PExPIn/Control System/Wf Controller/Controller/N1cSP Limit Controllers/N1 Max Controller ==
  Prelookup : Inport
  N1 : Inport  Port=2
  N1cCmd : Inport  Port=3
  Bus Selector : BusSelector  OutputSignals=k_Alt,f_Alt,k_MN,f_MN,k_PwrInLP,f_PwrInLP,k_PwrInHP,f_PwrInHP
  Constant : Constant  Value=MWS.Init.IC.N1c
  Constant1 : Constant  Value=MWS.Cntrl.WfCntrl.N1Max.SP
  Discrete-Time Integrator : DiscreteIntegrator  SampleTime=MWS.In.Ts  ICPrevOutput=DiscIntNeverNeededParam  ICPrevScaledInput=DiscIntNeverNeededParam
  Divide2 : Product  Inputs=**
  Divide3 : Product  Inputs=**
  Gain : Gain  Gain=MWS.Cntrl.WfCntrl.N1Max.Kiwp
  Ki Interpolation Using Prelookup : Interpolation_n-D  NumberOfTableDimensions=4  Table=MWS.Cntrl.WfCntrl.N1Max.Ki_array  InternalRulePriority=Speed
      settings: InputPortMap=u0,u1,u2,u3,u4,u5,u6,u7
  Kp Interpolation Using Prelookup : Interpolation_n-D  NumberOfTableDimensions=4  Table=MWS.Cntrl.WfCntrl.N1Max.Kp_array  InternalRulePriority=Speed
      settings: InputPortMap=u0,u1,u2,u3,u4,u5,u6,u7
  Sum : Sum  Inputs=|+-
  Sum1 : Sum  Inputs=|++
  Sum2 : Sum  Inputs=|-+
  Sum3 : Sum  Inputs=|+-
  Sum4 : Sum  Inputs=|++
  N1cDmd : Outport  VectorParamsAs1DForOutWhenUnconnected=off
  N1Max_SP : Outport  Port=2  VectorParamsAs1DForOutWhenUnconnected=off
  wires:
  N1/1 -> Sum/2
  Divide3/1 -> Sum1/1
  [Error] -> Divide3/2
  Sum1/1 -> Sum4/1
  Kp Interpolation Using Prelookup/1 -> Divide3/1  "Kp"
  [Error] -> Sum3/1
  Discrete-Time Integrator/1 -> Sum1/2
  Constant1/1 -> Sum/1, N1Max_SP/1  "N1_SP"
  Constant/1 -> Sum4/2
  Sum/1 -> [Error]
  Divide2/1 -> Discrete-Time Integrator/1
  Ki Interpolation Using Prelookup/1 -> Divide2/1  "Ki"
  Sum2/1 -> Gain/1
  N1cCmd/1 -> Sum2/1
  Gain/1 -> Sum3/2
  Sum4/1 -> Sum2/2, N1cDmd/1
  Sum3/1 -> Divide2/2
  Bus Selector/2 -> Ki Interpolation Using Prelookup/2, Kp Interpolation Using Prelookup/2  "<f_Alt>"
  Bus Selector/1 -> Ki Interpolation Using Prelookup/1, Kp Interpolation Using Prelookup/1  "<k_Alt>"
  Prelookup/1 -> Bus Selector/1
  Bus Selector/3 -> Ki Interpolation Using Prelookup/3, Kp Interpolation Using Prelookup/3  "<k_MN>"
  Bus Selector/4 -> Ki Interpolation Using Prelookup/4, Kp Interpolation Using Prelookup/4  "<f_MN>"
  Bus Selector/5 -> Ki Interpolation Using Prelookup/5, Kp Interpolation Using Prelookup/5  "<k_PwrInLP>"
  Bus Selector/6 -> Ki Interpolation Using Prelookup/6, Kp Interpolation Using Prelookup/6  "<f_PwrInLP>"
  Bus Selector/7 -> Ki Interpolation Using Prelookup/7, Kp Interpolation Using Prelookup/7  "<k_PwrInHP>"
  Bus Selector/8 -> Ki Interpolation Using Prelookup/8, Kp Interpolation Using Prelookup/8  "<f_PwrInHP>"

== system AGTF30SysDyn_PExPIn/Control System/Wf Controller/Controller/N1cSP Limit Controllers/N3 Max Controller ==
  Prelookup : Inport
  N3 : Inport  Port=2
  N1cCmd : Inport  Port=3
  Bus Selector : BusSelector  OutputSignals=k_Alt,f_Alt,k_MN,f_MN,k_PwrInLP,f_PwrInLP,k_PwrInHP,f_PwrInHP
  Constant : Constant  Value=MWS.Init.IC.N1c
  Constant1 : Constant  Value=MWS.Cntrl.WfCntrl.N3Max.SP
  Discrete-Time Integrator : DiscreteIntegrator  SampleTime=MWS.In.Ts  ICPrevOutput=DiscIntNeverNeededParam  ICPrevScaledInput=DiscIntNeverNeededParam
  Divide2 : Product  Inputs=**
  Divide3 : Product  Inputs=**
  Gain : Gain  Gain=MWS.Cntrl.WfCntrl.N3Max.Kiwp
  Ki Interpolation Using Prelookup : Interpolation_n-D  NumberOfTableDimensions=4  Table=MWS.Cntrl.WfCntrl.N3Max.Ki_array  InternalRulePriority=Speed
      settings: InputPortMap=u0,u1,u2,u3,u4,u5,u6,u7
  Kp Interpolation Using Prelookup : Interpolation_n-D  NumberOfTableDimensions=4  Table=MWS.Cntrl.WfCntrl.N3Max.Kp_array  InternalRulePriority=Speed
      settings: InputPortMap=u0,u1,u2,u3,u4,u5,u6,u7
  Sum : Sum  Inputs=|+-
  Sum1 : Sum  Inputs=|++
  Sum2 : Sum  Inputs=|-+
  Sum3 : Sum  Inputs=|+-
  Sum4 : Sum  Inputs=|++
  N1cDmd : Outport  VectorParamsAs1DForOutWhenUnconnected=off
  N3Max_SP : Outport  Port=2  VectorParamsAs1DForOutWhenUnconnected=off
  wires:
  Sum3/1 -> Divide2/2
  Ki Interpolation Using Prelookup/1 -> Divide2/1  "Ki"
  Divide2/1 -> Discrete-Time Integrator/1
  Sum/1 -> [Error]
  Constant/1 -> Sum4/2
  Constant1/1 -> N3Max_SP/1, Sum/1  "N3_SP"
  Discrete-Time Integrator/1 -> Sum1/2
  [Error] -> Sum3/1
  Kp Interpolation Using Prelookup/1 -> Divide3/1  "Kp"
  Sum1/1 -> Sum4/1
  [Error] -> Divide3/2
  Divide3/1 -> Sum1/1
  N3/1 -> Sum/2
  Sum4/1 -> Sum2/2, N1cDmd/1
  Gain/1 -> Sum3/2
  N1cCmd/1 -> Sum2/1
  Sum2/1 -> Gain/1
  Bus Selector/2 -> Ki Interpolation Using Prelookup/2, Kp Interpolation Using Prelookup/2  "<f_Alt>"
  Bus Selector/1 -> Ki Interpolation Using Prelookup/1, Kp Interpolation Using Prelookup/1  "<k_Alt>"
  Prelookup/1 -> Bus Selector/1
  Bus Selector/3 -> Ki Interpolation Using Prelookup/3, Kp Interpolation Using Prelookup/3  "<k_MN>"
  Bus Selector/4 -> Ki Interpolation Using Prelookup/4, Kp Interpolation Using Prelookup/4  "<f_MN>"
  Bus Selector/5 -> Ki Interpolation Using Prelookup/5, Kp Interpolation Using Prelookup/5  "<k_PwrInLP>"
  Bus Selector/6 -> Ki Interpolation Using Prelookup/6, Kp Interpolation Using Prelookup/6  "<f_PwrInLP>"
  Bus Selector/7 -> Ki Interpolation Using Prelookup/7, Kp Interpolation Using Prelookup/7  "<k_PwrInHP>"
  Bus Selector/8 -> Ki Interpolation Using Prelookup/8, Kp Interpolation Using Prelookup/8  "<f_PwrInHP>"

== system AGTF30SysDyn_PExPIn/Control System/Wf Controller/Controller/N1cSP Limit Controllers/Ps3 Max Controller ==
  Prelookup : Inport
  Ps3 : Inport  Port=2
  N1cCmd : Inport  Port=3
  Bus Selector : BusSelector  OutputSignals=k_Alt,f_Alt,k_MN,f_MN,k_PwrInLP,f_PwrInLP,k_PwrInHP,f_PwrInHP
  Constant : Constant  Value=MWS.Init.IC.N1c
  Constant1 : Constant  Value=MWS.Cntrl.WfCntrl.Ps3Max.SP
  Discrete-Time Integrator : DiscreteIntegrator  SampleTime=MWS.In.Ts  ICPrevOutput=DiscIntNeverNeededParam  ICPrevScaledInput=DiscIntNeverNeededParam
  Divide2 : Product  Inputs=**
  Divide3 : Product  Inputs=**
  Gain : Gain  Gain=MWS.Cntrl.WfCntrl.Ps3Max.Kiwp
  Ki Interpolation Using Prelookup : Interpolation_n-D  NumberOfTableDimensions=4  Table=MWS.Cntrl.WfCntrl.Ps3Max.Ki_array  InternalRulePriority=Speed
      settings: InputPortMap=u0,u1,u2,u3,u4,u5,u6,u7
  Kp Interpolation Using Prelookup : Interpolation_n-D  NumberOfTableDimensions=4  Table=MWS.Cntrl.WfCntrl.Ps3Max.Kp_array  InternalRulePriority=Speed
      settings: InputPortMap=u0,u1,u2,u3,u4,u5,u6,u7
  Sum : Sum  Inputs=|+-
  Sum1 : Sum  Inputs=|++
  Sum2 : Sum  Inputs=|-+
  Sum3 : Sum  Inputs=|+-
  Sum4 : Sum  Inputs=|++
  N1cDmd : Outport  VectorParamsAs1DForOutWhenUnconnected=off
  Ps3Max_SP : Outport  Port=2  VectorParamsAs1DForOutWhenUnconnected=off
  wires:
  Divide3/1 -> Sum1/1
  [Error] -> Divide3/2
  Sum1/1 -> Sum4/1
  Kp Interpolation Using Prelookup/1 -> Divide3/1  "Kp"
  [Error] -> Sum3/1
  Discrete-Time Integrator/1 -> Sum1/2
  Constant/1 -> Sum4/2
  Divide2/1 -> Discrete-Time Integrator/1
  Ki Interpolation Using Prelookup/1 -> Divide2/1  "Ki"
  Ps3/1 -> Sum/2
  Constant1/1 -> Ps3Max_SP/1, Sum/1  "Ps3_SP"
  Sum/1 -> [Error]
  Sum2/1 -> Gain/1
  N1cCmd/1 -> Sum2/1
  Gain/1 -> Sum3/2
  Sum4/1 -> Sum2/2, N1cDmd/1
  Sum3/1 -> Divide2/2
  Bus Selector/2 -> Ki Interpolation Using Prelookup/2, Kp Interpolation Using Prelookup/2  "<f_Alt>"
  Bus Selector/1 -> Ki Interpolation Using Prelookup/1, Kp Interpolation Using Prelookup/1  "<k_Alt>"
  Prelookup/1 -> Bus Selector/1
  Bus Selector/3 -> Ki Interpolation Using Prelookup/3, Kp Interpolation Using Prelookup/3  "<k_MN>"
  Bus Selector/4 -> Ki Interpolation Using Prelookup/4, Kp Interpolation Using Prelookup/4  "<f_MN>"
  Bus Selector/5 -> Ki Interpolation Using Prelookup/5, Kp Interpolation Using Prelookup/5  "<k_PwrInLP>"
  Bus Selector/6 -> Ki Interpolation Using Prelookup/6, Kp Interpolation Using Prelookup/6  "<f_PwrInLP>"
  Bus Selector/7 -> Ki Interpolation Using Prelookup/7, Kp Interpolation Using Prelookup/7  "<k_PwrInHP>"
  Bus Selector/8 -> Ki Interpolation Using Prelookup/8, Kp Interpolation Using Prelookup/8  "<f_PwrInHP>"

== system AGTF30SysDyn_PExPIn/Control System/Wf Controller/Controller/N1cSP Limit Controllers/Ps3 Min Controller ==
  Prelookup : Inport
  Ps3 : Inport  Port=2
  N1cCmd : Inport  Port=3
  Bus Selector : BusSelector  OutputSignals=k_Alt,f_Alt,k_MN,f_MN,k_PwrInLP,f_PwrInLP,k_PwrInHP,f_PwrInHP,k_PwrInHP_Ps3Min,f_PwrInHP_Ps3Min
  Constant : Constant  Value=MWS.Init.IC.N1c
  Discrete-Time Integrator : DiscreteIntegrator  SampleTime=MWS.In.Ts  ICPrevOutput=DiscIntNeverNeededParam  ICPrevScaledInput=DiscIntNeverNeededParam
  Divide2 : Product  Inputs=**
  Divide3 : Product  Inputs=**
  Gain : Gain  Gain=MWS.Cntrl.WfCntrl.Ps3Min.Kiwp
  Ki Interpolation Using Prelookup : Interpolation_n-D  NumberOfTableDimensions=3  Table=MWS.Cntrl.WfCntrl.Ps3Min.Ki_array  InternalRulePriority=Speed
      settings: InputPortMap=u0,u1,u2,u3,u4,u5
  Kp Interpolation Using Prelookup : Interpolation_n-D  NumberOfTableDimensions=3  Table=MWS.Cntrl.WfCntrl.Ps3Min.Kp_array  InternalRulePriority=Speed
      settings: InputPortMap=u0,u1,u2,u3,u4,u5
  Ps3minSP Interpolation Using Prelookup : Interpolation_n-D  NumberOfTableDimensions=4  Table=MWS.Cntrl.WfCntrl.Sched.Ps3MinSP.Ps3MinSP_array  InternalRulePriority=Speed
      settings: InputPortMap=u0,u1,u2,u3,u4,u5,u6,u7
  Sum : Sum  Inputs=|+-
  Sum1 : Sum  Inputs=|++
  Sum2 : Sum  Inputs=|-+
  Sum3 : Sum  Inputs=|+-
  Sum4 : Sum  Inputs=|++
  N1cDmd : Outport  VectorParamsAs1DForOutWhenUnconnected=off
  Ps3Min_SP : Outport  Port=2  VectorParamsAs1DForOutWhenUnconnected=off
  wires:
  Sum3/1 -> Divide2/2
  Ki Interpolation Using Prelookup/1 -> Divide2/1  "Ki"
  Divide2/1 -> Discrete-Time Integrator/1
  Sum/1 -> [Error]
  Constant/1 -> Sum4/2
  Ps3minSP Interpolation Using Prelookup/1 -> Ps3Min_SP/1, Sum/1  "Ps3min_SP"
  Discrete-Time Integrator/1 -> Sum1/2
  [Error] -> Sum3/1
  Kp Interpolation Using Prelookup/1 -> Divide3/1  "Kp"
  Sum1/1 -> Sum4/1
  [Error] -> Divide3/2
  Divide3/1 -> Sum1/1
  Ps3/1 -> Sum/2
  Sum4/1 -> Sum2/2, N1cDmd/1
  Sum2/1 -> Gain/1
  N1cCmd/1 -> Sum2/1
  Gain/1 -> Sum3/2
  Bus Selector/5 -> Ps3minSP Interpolation Using Prelookup/5  "<k_PwrInLP>"
  Bus Selector/2 -> Ki Interpolation Using Prelookup/2, Kp Interpolation Using Prelookup/2, Ps3minSP Interpolation Using Prelookup/2  "<f_Alt>"
  Bus Selector/1 -> Ps3minSP Interpolation Using Prelookup/1, Ki Interpolation Using Prelookup/1, Kp Interpolation Using Prelookup/1  "<k_Alt>"
  Bus Selector/6 -> Ps3minSP Interpolation Using Prelookup/6  "<f_PwrInLP>"
  Prelookup/1 -> Bus Selector/1
  Bus Selector/3 -> Ki Interpolation Using Prelookup/3, Kp Interpolation Using Prelookup/3, Ps3minSP Interpolation Using Prelookup/3  "<k_MN>"
  Bus Selector/4 -> Ki Interpolation Using Prelookup/4, Kp Interpolation Using Prelookup/4, Ps3minSP Interpolation Using Prelookup/4  "<f_MN>"
  Bus Selector/7 -> Ps3minSP Interpolation Using Prelookup/7  "<k_PwrInHP>"
  Bus Selector/8 -> Ps3minSP Interpolation Using Prelookup/8  "<f_PwrInHP>"
  Bus Selector/9 -> Ki Interpolation Using Prelookup/5, Kp Interpolation Using Prelookup/5  "<k_PwrInHP_Ps3Min>"
  Bus Selector/10 -> Ki Interpolation Using Prelookup/6, Kp Interpolation Using Prelookup/6  "<f_PwrInHP_Ps3Min>"

== system AGTF30SysDyn_PExPIn/Control System/Wf Controller/Controller/N1cSP Limit Controllers/T3 Max Controller ==
  Prelookup : Inport
  T3 : Inport  Port=2
  N1cCmd : Inport  Port=3
  Bus Selector : BusSelector  OutputSignals=k_Alt,f_Alt,k_MN,f_MN,k_PwrInLP,f_PwrInLP,k_PwrInHP,f_PwrInHP
  Constant : Constant  Value=MWS.Init.IC.N1c
  Constant1 : Constant  Value=MWS.Cntrl.WfCntrl.T3Max.SP
  Discrete-Time Integrator : DiscreteIntegrator  SampleTime=MWS.In.Ts  ICPrevOutput=DiscIntNeverNeededParam  ICPrevScaledInput=DiscIntNeverNeededParam
  Divide2 : Product  Inputs=**
  Divide3 : Product  Inputs=**
  Gain : Gain  Gain=MWS.Cntrl.WfCntrl.T3Max.Kiwp
  Ki Interpolation Using Prelookup : Interpolation_n-D  NumberOfTableDimensions=4  Table=MWS.Cntrl.WfCntrl.T3Max.Ki_array  InternalRulePriority=Speed
      settings: InputPortMap=u0,u1,u2,u3,u4,u5,u6,u7
  Kp Interpolation Using Prelookup : Interpolation_n-D  NumberOfTableDimensions=4  Table=MWS.Cntrl.WfCntrl.T3Max.Kp_array  InternalRulePriority=Speed
      settings: InputPortMap=u0,u1,u2,u3,u4,u5,u6,u7
  Sum : Sum  Inputs=|+-
  Sum1 : Sum  Inputs=|++
  Sum2 : Sum  Inputs=|-+
  Sum3 : Sum  Inputs=|+-
  Sum4 : Sum  Inputs=|++
  N1cDmd : Outport  VectorParamsAs1DForOutWhenUnconnected=off
  T3Max_SP : Outport  Port=2  VectorParamsAs1DForOutWhenUnconnected=off
  wires:
  Divide3/1 -> Sum1/1
  [Error] -> Divide3/2
  Sum1/1 -> Sum4/1
  Sum4/1 -> Sum2/2, N1cDmd/1
  Kp Interpolation Using Prelookup/1 -> Divide3/1  "Kp"
  [Error] -> Sum3/1
  Discrete-Time Integrator/1 -> Sum1/2
  Constant/1 -> Sum4/2
  Divide2/1 -> Discrete-Time Integrator/1
  Ki Interpolation Using Prelookup/1 -> Divide2/1  "Ki"
  Sum3/1 -> Divide2/2
  T3/1 -> Sum/2
  Constant1/1 -> T3Max_SP/1, Sum/1  "T3_SP"
  Sum/1 -> [Error]
  N1cCmd/1 -> Sum2/1
  Sum2/1 -> Gain/1
  Gain/1 -> Sum3/2
  Prelookup/1 -> Bus Selector/1
  Bus Selector/1 -> Ki Interpolation Using Prelookup/1, Kp Interpolation Using Prelookup/1  "<k_Alt>"
  Bus Selector/2 -> Ki Interpolation Using Prelookup/2, Kp Interpolation Using Prelookup/2  "<f_Alt>"
  Bus Selector/3 -> Ki Interpolation Using Prelookup/3, Kp Interpolation Using Prelookup/3  "<k_MN>"
  Bus Selector/4 -> Ki Interpolation Using Prelookup/4, Kp Interpolation Using Prelookup/4  "<f_MN>"
  Bus Selector/5 -> Ki Interpolation Using Prelookup/5, Kp Interpolation Using Prelookup/5  "<k_PwrInLP>"
  Bus Selector/6 -> Ki Interpolation Using Prelookup/6, Kp Interpolation Using Prelookup/6  "<f_PwrInLP>"
  Bus Selector/7 -> Ki Interpolation Using Prelookup/7, Kp Interpolation Using Prelookup/7  "<k_PwrInHP>"
  Bus Selector/8 -> Ki Interpolation Using Prelookup/8, Kp Interpolation Using Prelookup/8  "<f_PwrInHP>"

== system AGTF30SysDyn_PExPIn/Control System/Wf Controller/Controller/N1cSP Limit Controllers/T4 Max Controller ==
  Prelookup : Inport
  T4 : Inport  Port=2
  N1cCmd : Inport  Port=3
  Bus Selector : BusSelector  OutputSignals=k_Alt,f_Alt,k_MN,f_MN,k_PwrInLP,f_PwrInLP,k_PwrInHP,f_PwrInHP
  Constant : Constant  Value=MWS.Init.IC.N1c
  Constant7 : Constant  Value=MWS.Cntrl.WfCntrl.T4Max.SP
  Discrete-Time Integrator : DiscreteIntegrator  SampleTime=MWS.In.Ts  ICPrevOutput=DiscIntNeverNeededParam  ICPrevScaledInput=DiscIntNeverNeededParam
  Divide2 : Product  Inputs=**
  Divide3 : Product  Inputs=**
  Gain : Gain  Gain=MWS.Cntrl.WfCntrl.T4Max.Kiwp
  Ki Interpolation Using Prelookup : Interpolation_n-D  NumberOfTableDimensions=4  Table=MWS.Cntrl.WfCntrl.T4Max.Ki_array  InternalRulePriority=Speed
      settings: InputPortMap=u0,u1,u2,u3,u4,u5,u6,u7
  Kp Interpolation Using Prelookup : Interpolation_n-D  NumberOfTableDimensions=4  Table=MWS.Cntrl.WfCntrl.T4Max.Kp_array  InternalRulePriority=Speed
      settings: InputPortMap=u0,u1,u2,u3,u4,u5,u6,u7
  Sum : Sum  Inputs=|+-
  Sum1 : Sum  Inputs=|++
  Sum2 : Sum  Inputs=|-+
  Sum3 : Sum  Inputs=|+-
  Sum4 : Sum  Inputs=|++
  N1cDmd : Outport  VectorParamsAs1DForOutWhenUnconnected=off
  T4Max_SP : Outport  Port=2  VectorParamsAs1DForOutWhenUnconnected=off
  wires:
  Ki Interpolation Using Prelookup/1 -> Divide2/1  "Ki"
  Divide2/1 -> Discrete-Time Integrator/1
  Sum/1 -> [Error]
  Constant/1 -> Sum4/2
  Constant7/1 -> Sum/1, T4Max_SP/1  "T4_SP"
  Discrete-Time Integrator/1 -> Sum1/2
  [Error] -> Sum3/1
  Kp Interpolation Using Prelookup/1 -> Divide3/1  "Kp"
  Sum1/1 -> Sum4/1
  [Error] -> Divide3/2
  Divide3/1 -> Sum1/1
  T4/1 -> Sum/2
  Sum2/1 -> Gain/1
  N1cCmd/1 -> Sum2/1
  Gain/1 -> Sum3/2
  Sum4/1 -> Sum2/2, N1cDmd/1
  Sum3/1 -> Divide2/2
  Prelookup/1 -> Bus Selector/1
  Bus Selector/2 -> Ki Interpolation Using Prelookup/2, Kp Interpolation Using Prelookup/2  "<f_Alt>"
  Bus Selector/1 -> Ki Interpolation Using Prelookup/1, Kp Interpolation Using Prelookup/1  "<k_Alt>"
  Bus Selector/3 -> Ki Interpolation Using Prelookup/3, Kp Interpolation Using Prelookup/3  "<k_MN>"
  Bus Selector/4 -> Ki Interpolation Using Prelookup/4, Kp Interpolation Using Prelookup/4  "<f_MN>"
  Bus Selector/5 -> Ki Interpolation Using Prelookup/5, Kp Interpolation Using Prelookup/5  "<k_PwrInLP>"
  Bus Selector/6 -> Ki Interpolation Using Prelookup/6, Kp Interpolation Using Prelookup/6  "<f_PwrInLP>"
  Bus Selector/7 -> Ki Interpolation Using Prelookup/7, Kp Interpolation Using Prelookup/7  "<k_PwrInHP>"
  Bus Selector/8 -> Ki Interpolation Using Prelookup/8, Kp Interpolation Using Prelookup/8  "<f_PwrInHP>"

== system AGTF30SysDyn_PExPIn/Control System/Wf Controller/Controller/N1cSP Limit Controllers/T45 Max Controller ==
  Prelookup : Inport
  T45 : Inport  Port=2
  N1cCmd : Inport  Port=3
  Bus Selector : BusSelector  OutputSignals=k_Alt,f_Alt,k_MN,f_MN,k_PwrInLP,f_PwrInLP,k_PwrInHP,f_PwrInHP
  Constant : Constant  Value=MWS.Init.IC.N1c
  Discrete-Time Integrator : DiscreteIntegrator  SampleTime=MWS.In.Ts  ICPrevOutput=DiscIntNeverNeededParam  ICPrevScaledInput=DiscIntNeverNeededParam
  Divide2 : Product  Inputs=**
  Divide3 : Product  Inputs=**
  Gain : Gain  Gain=MWS.Cntrl.WfCntrl.T45Max.Kiwp
  Ki Interpolation Using Prelookup : Interpolation_n-D  NumberOfTableDimensions=4  Table=MWS.Cntrl.WfCntrl.T45Max.Ki_array  InternalRulePriority=Speed
      settings: InputPortMap=u0,u1,u2,u3,u4,u5,u6,u7
  Kp Interpolation Using Prelookup : Interpolation_n-D  NumberOfTableDimensions=4  Table=MWS.Cntrl.WfCntrl.T45Max.Kp_array  InternalRulePriority=Speed
      settings: InputPortMap=u0,u1,u2,u3,u4,u5,u6,u7
  Sum : Sum  Inputs=|+-
  Sum1 : Sum  Inputs=|++
  Sum2 : Sum  Inputs=|-+
  Sum3 : Sum  Inputs=|+-
  Sum4 : Sum  Inputs=|++
  T45 Max Set-Point Interpolation Using Prelookup : Interpolation_n-D  NumberOfTableDimensions=4  Table=MWS.Cntrl.WfCntrl.Sched.T45MaxSP.T45MaxSP_array  InternalRulePriority=Speed
      settings: InputPortMap=u0,u1,u2,u3,u4,u5,u6,u7
  N1cDmd : Outport  VectorParamsAs1DForOutWhenUnconnected=off
  T4Max_SP : Outport  Port=2  VectorParamsAs1DForOutWhenUnconnected=off
  wires:
  Prelookup/1 -> Bus Selector/1
  Sum3/1 -> Divide2/2
  Sum4/1 -> N1cDmd/1, Sum2/2
  Gain/1 -> Sum3/2
  N1cCmd/1 -> Sum2/1
  Sum2/1 -> Gain/1
  T45/1 -> Sum/2
  Divide3/1 -> Sum1/1
  [Error] -> Divide3/2
  Sum1/1 -> Sum4/1
  Kp Interpolation Using Prelookup/1 -> Divide3/1  "Kp"
  [Error] -> Sum3/1
  Discrete-Time Integrator/1 -> Sum1/2
  T45 Max Set-Point Interpolation Using Prelookup/1 -> Sum/1, T4Max_SP/1  "T5_SP"
  Constant/1 -> Sum4/2
  Sum/1 -> [Error]
  Divide2/1 -> Discrete-Time Integrator/1
  Ki Interpolation Using Prelookup/1 -> Divide2/1  "Ki"
  Bus Selector/1 -> Ki Interpolation Using Prelookup/1, Kp Interpolation Using Prelookup/1, T45 Max Set-Point Interpolation Using Prelookup/1  "<k_Alt>"
  Bus Selector/2 -> Ki Interpolation Using Prelookup/2, Kp Interpolation Using Prelookup/2, T45 Max Set-Point Interpolation Using Prelookup/2  "<f_Alt>"
  Bus Selector/3 -> Kp Interpolation Using Prelookup/3, Ki Interpolation Using Prelookup/3, T45 Max Set-Point Interpolation Using Prelookup/3  "<k_MN>"
  Bus Selector/4 -> Kp Interpolation Using Prelookup/4, Ki Interpolation Using Prelookup/4, T45 Max Set-Point Interpolation Using Prelookup/4  "<f_MN>"
  Bus Selector/5 -> Ki Interpolation Using Prelookup/5, Kp Interpolation Using Prelookup/5, T45 Max Set-Point Interpolation Using Prelookup/5  "<k_PwrInLP>"
  Bus Selector/6 -> Ki Interpolation Using Prelookup/6, Kp Interpolation Using Prelookup/6, T45 Max Set-Point Interpolation Using Prelookup/6  "<f_PwrInLP>"
  Bus Selector/7 -> Ki Interpolation Using Prelookup/7, Kp Interpolation Using Prelookup/7, T45 Max Set-Point Interpolation Using Prelookup/7  "<k_PwrInHP>"
  Bus Selector/8 -> Ki Interpolation Using Prelookup/8, Kp Interpolation Using Prelookup/8, T45 Max Set-Point Interpolation Using Prelookup/8  "<f_PwrInHP>"
